simulink model "A1d"  (R2025b)
settings: Solver=FixedStepAuto  StartTime=0.0  StopTime=20  FixedStep=0.001  RelTol=1e-3
values from neighbouring files (symbols this model uses):
  k1 = (m*l)/(m*l^2+J)    (= 1.25)    [Lab1.m]
  k2 = (m*g*l)/(m*l^2+J)    (= 12.2625)    [Lab1.m]
  k3 = (c_r)/(m*l^2+J)    (= 0.3125)    [Lab1.m]
  u0 = 10    [Lab1.m]
undefined symbols (not defined in the file or in its folder): A, b, c, d
settings Model: Creator=david  LastModifiedBy=david

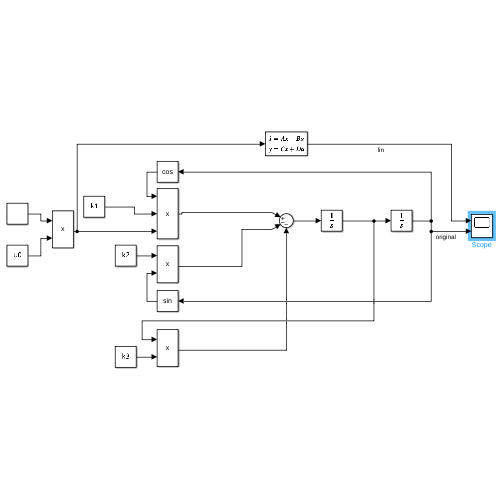
[thumbnail: Simulink's stored preview of the top-level diagram]
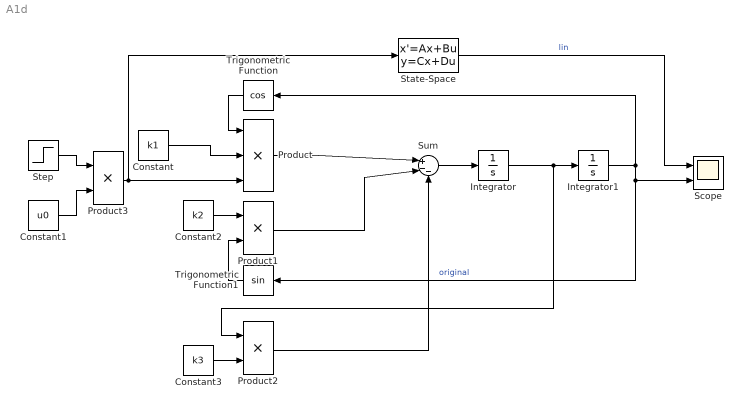
== system A1d ==
  Constant : Constant  Value=k1
  Constant1 : Constant  Value=u0
  Constant2 : Constant  Value=k2
  Constant3 : Constant  Value=k3
  Integrator : Integrator
  Integrator1 : Integrator
  Product : Product  Inputs=3
  Product1 : Product
  Product2 : Product
  Product3 : Product
  Scope : Scope  NumInputPorts=2
      settings: ActiveDisplayYMinimum=0.27120843198256317  ActiveDisplayYMaximum=20.605221363784302
  State-Space : StateSpace  A=A  B=b  C=c  D=d  InitialCondition=0
  Step : Step  SampleTime=0
  Sum : Sum  Inputs=|+--
  Trigonometric Function : Trigonometry  Operator=cos
  Trigonometric Function1 : Trigonometry
  wires:
  Integrator/1 -> Product2/1, Integrator1/1
  Integrator1/1 -> Scope/2, Trigonometric Function1/1, Trigonometric Function/1  "original"
  Constant/1 -> Product/2
  Product3/1 -> State-Space/1, Product/3
  Trigonometric Function/1 -> Product/1
  Product/1 -> Sum/1
  Constant2/1 -> Product1/1
  Trigonometric Function1/1 -> Product1/2
  Product1/1 -> Sum/2
  Product2/1 -> Sum/3
  Constant3/1 -> Product2/2
  Sum/1 -> Integrator/1
  Step/1 -> Product3/1
  Constant1/1 -> Product3/2
  State-Space/1 -> Scope/1  "lin"
